simulink model "pend2"  (Simulink 6.6)
settings: Solver=ode45  StartTime=0.0  StopTime=7  MaxStep=0.04  RelTol=1e-3
undefined symbols (not defined in the file): pend2_control
settings Model: Creator=nsz  LastModifiedBy=nsz  ExtModeAutoUpdateStatusClock=off

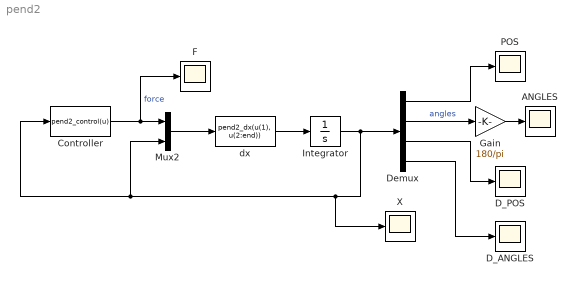
== system pend2 ==
  ANGLES : Scope
      settings: YMin=-15  YMax=27.5  SaveName=ScopeData2
  Controller : MATLABFcn  MATLABFcn=pend2_control(u)  OutputDimensions=1
  D_ANGLES : Scope
      settings: YMin=-3.75  YMax=2  SaveName=ScopeData4
  D_POS : Scope
      settings: YMin=-3.75  YMax=2  SaveName=ScopeData3
  Demux : Demux  Outputs=[1 2 1 2]
  F : Scope
      settings: YMin=0.01  YMax=0.07  SaveName=ScopeData5
  Gain : Gain  Gain=180/pi
  Integrator : Integrator  InitialCondition=[0 5*pi/180 -5*pi/180 0 0 0]
  Mux2 : Mux  Inputs=2
  POS : Scope
      settings: YMin=-3.75  YMax=2
  X : Scope
      settings: YMin=-3.75  YMax=2
  dx : MATLABFcn  MATLABFcn=pend2_dx(u(1), u(2:end))  OutputDimensions=6
  wires:
  Mux2/1 -> dx/1
  Controller/1 -> Mux2/1, F/1  "force"
  Integrator/1 -> Controller/1, Mux2/2, X/1, Demux/1
  Demux/1 -> POS/1
  Demux/2 -> Gain/1  "angles"
  Demux/3 -> D_POS/1
  Demux/4 -> D_ANGLES/1
  dx/1 -> Integrator/1
  Gain/1 -> ANGLES/1
